simulink model "trackTwoSimulinkPerformanceTest"  (R2014b)
settings: Solver=FixedStepDiscrete  StartTime=0.0  StopTime=inf  RelTol=1e-3
InitFcn:
  | threshold = initTrackTwoMinions(debugFlag);
undefined symbols (not defined in the file or in its folder): IsPositionTracked, IsSkeletonTracked, JointDepthIndices, JointImageIndices, JointTrackingState, JointWorldCoordinates, none, PositionDepthIndices, PositionImageIndices, PositionWorldCoordinates, SegmentationData, SkeletonTrackingID, videoinput
libraries: visionsinks x3, visiontextngfix x1, imaqlib x1
settings Model: Creator=gsalhotr  LastModifiedBy=gsalhotr

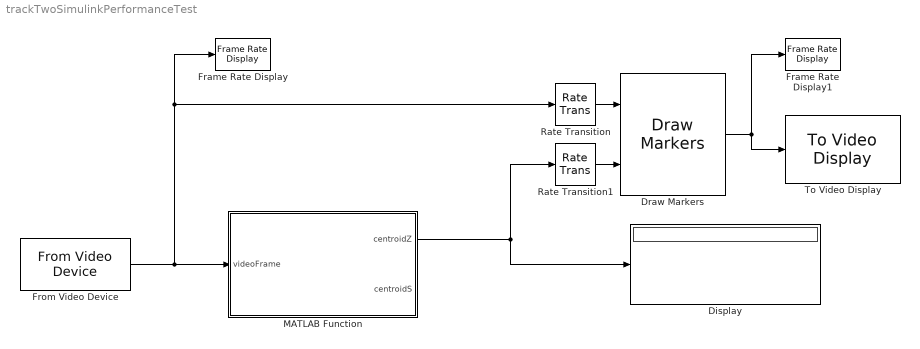
== system trackTwoSimulinkPerformanceTest ==
  Display : Display
  Draw Markers : visiontextngfix/Draw Markers  shape=X-mark  size=10  fill=off  fillClrSource=Specify via dialog  display=User-specified value  intensity=200  color=[255 0 0]  opacity=0.6  viewport=Entire image  antialiasing=off  inType=Obsolete  imagePorts=One multidimensional signal  prodOutputMode=Binary point scaling  prodOutputWordLength=32  prodOutputFracLength=14  memoryMode=Specify word length  memoryWordLength=16  memoryFracLength=15  roundingMode=Floor  overflowMode=off
  Frame Rate Display : visionsinks/Frame Rate Display  UpdateRate=10
  Frame Rate Display1 : visionsinks/Frame Rate Display  UpdateRate=10
  From Video Device : imaqlib/From Video Device  DeviceMenu=winvideo 1 (USB Video Device)  Device=winvideo 1 (USB Video Device)  ObjConstructor=videoinput('winvideo', 1)  VideoFormatMenu=MJPG_640x480  VideoFormat=MJPG_640x480  VideoSource=input1  ROIPosition=[0 0 480 640]  EnableHWTrigger=off  TriggerConfiguration=none/none  SampleTime=1/30  OutputPortsMode=One multidimensional signal  DataType=single  CanDoHWTrigger=no  ReturnedColorSpace=rgb  BlockHandle=1921.0006  ROIWidth=640  ROIHeight=480  ROIColumn=0  ROIRow=0  EngXMLPath=C:\Program Files\MATLAB\R2014b\toolbox\imaq\imaq\private  DevXMLPath=C:\MATLAB\SupportPackages\R2014b\osgenericvideointerface\toolbox\imaq\supportpackages\genericvideo\adaptor\win64  EngLibPath=C:\Program Files\MATLAB\R2014b\toolbox\imaq\imaqblks\imaqmex\win64  ColorSpace=rgb  BayerSensorAlignment=grbg  AllMetadata=IsPositionTracked;IsSkeletonTracked;JointDepthIndices;JointImageIndices;JointTrackingState;JointWorldCoordinates;PositionDepthIndices;PositionImageIndices;PositionWorldCoordinates;SegmentationData;SkeletonTrackingID
  MATLAB Function : MATLAB Function  TreatAsAtomicUnit=on
  Rate Transition : RateTransition  OutPortSampleTime=0.5
  Rate Transition1 : RateTransition  OutPortSampleTime=0.5
  To Video Display : visionsinks/To Video Display  inputType=Obsolete  imagePorts=One multidimensional signal  OutputDevice=On-screen video monitor  fullScreen=off  videoWindowX=884  videoWindowY=-1  saveWindowSize=off  videoWindowWidth=640  videoWindowHeight=480  dataOrg=Column-major  openAtMdlStart=on  isWindowOpen=on  inputColorFormat=RGB
  wires:
  From Video Device/1 -> Frame Rate Display/1, Rate Transition/1, MATLAB Function/1(videoFrame)
  Draw Markers/1 -> To Video Display/1, Frame Rate Display1/1
  Rate Transition/1 -> Draw Markers/1
  MATLAB Function/1(centroidZ) -> Display/1, Rate Transition1/1
  Rate Transition1/1 -> Draw Markers/2

== matlab function trackTwoSimulinkPerformanceTest/MATLAB Function ==
  data: videoFrame input; centroidZ output; centroidS output
function [centroidZ,centroidS] = fcn(videoFrame)
%#codegen
    coder.extrinsic('trackTwoMinions');
    
    centroidZ = zeros([2,2],'single');
    centroidS = zeros([1,2],'double');
    [centroidZ,centroidS] = trackTwoMinions(videoFrame,0);
end
